simulink model "ctrl_TAPM_2015"  (R2015a)
settings: Solver=ode3  StartTime=0.0  StopTime=inf  FixedStep=0.01  RelTol=1e-3
undefined symbols (not defined in the file): C, D, DiscIntNeverNeededParam, eps_c, epsilon, hd, hd2, I_s, k_cc, K_omega, K_q1f, K_q1r, K_q2f, K_q2r, K_q3f, K_q3r, K_q4f, K_q4r, K_q5f, K_q5r, K_q6f, K_q6r, K_T1f, K_T1r, K_T2f, K_T2r, K_T3f, K_T3r, K_T4f, K_T4r, K_T5f, K_T5r, K_T6f, K_T6r, Kp, Max_Acceleration, Max_rotation, Max_thrust, Min_thrust, n_c, n_max, p_cc, pwm_thr1_backward, pwm_thr1_forward, pwm_thr2_backward, pwm_thr2_forward, pwm_thr3_backward, pwm_thr3_forward, pwm_thr4_backward, pwm_thr4_forward, pwm_thr5_backward, pwm_thr5_forward, pwm_thr6_backward, pwm_thr6_forward, Q_f0, Q_max, r_cc, Rho, Thruster
libraries: marine_gnc x10, dspstat3 x8, simulink x6, simulink_extras x3
(part 5 of 7)

== system ctrl_TAPM_2015/Thruster control /Thruster 3 ==
  Desired thrust 1 : Inport
  shaft speed : Inport  Port=2
  Constant : Constant  Value=hd2.den{1,1}
  Constant1 : Constant  Value=hd2.num{1,1}
  Delay : Delay  DelayLength=1  InitialCondition=0
  Discrete Transfer Fcn : DiscreteTransferFcn  NumeratorSource=Input port  DenominatorSource=Input port  Denominator=[0.2 1]  SampleTime=0.01  a0EqualsOne=on
      settings: InputPortMap=u0,p1,p3
  Losses (placeholder) : Constant  Value=0
  Propeller Hydrodynamics : Subsystem
  Shaft dynamics : Subsystem
  Thruster control : Subsystem
  "Commanded thrust " : Outport
  Shaft speed : Outport  Port=2
  wires:
  Losses (placeholder)/1 -> Propeller Hydrodynamics/1(env)
  Shaft dynamics/1(n) -> Propeller Hydrodynamics/2(n), Shaft speed/1
  Propeller Hydrodynamics/2(Qa) -> Delay/1
  Thruster control/1(Qc) -> Discrete Transfer Fcn/1
  Discrete Transfer Fcn/1 -> Shaft dynamics/1(Qm)
  Desired thrust 1/1 -> Thruster control/1("T_d ")
  Propeller Hydrodynamics/1(Ta) -> "Commanded thrust "/1
  Constant1/1 -> Discrete Transfer Fcn/2
  Constant/1 -> Discrete Transfer Fcn/3
  shaft speed/1 -> Thruster control/2(n)
  Delay/1 -> Shaft dynamics/2(Qa)

== system ctrl_TAPM_2015/Thruster control /Thruster 4 ==
  Desired thrust 1 : Inport
  shaft speed : Inport  Port=2
  Constant : Constant  Value=hd2.den{1,1}
  Constant1 : Constant  Value=hd2.num{1,1}
  Delay : Delay  DelayLength=1  InitialCondition=0
  Discrete Transfer Fcn : DiscreteTransferFcn  NumeratorSource=Input port  DenominatorSource=Input port  Denominator=[0.2 1]  SampleTime=0.01  a0EqualsOne=on
      settings: InputPortMap=u0,p1,p3
  Losses (placeholder) : Constant  Value=0
  Propeller Hydrodynamics : Subsystem
  Shaft dynamics : Subsystem
  Thruster control : Subsystem
  "Commanded thrust " : Outport
  Shaft speed : Outport  Port=2
  wires:
  Losses (placeholder)/1 -> Propeller Hydrodynamics/1(env)
  Shaft dynamics/1(n) -> Propeller Hydrodynamics/2(n), Shaft speed/1
  Propeller Hydrodynamics/2(Qa) -> Delay/1
  Thruster control/1(Qc) -> Discrete Transfer Fcn/1
  Discrete Transfer Fcn/1 -> Shaft dynamics/1(Qm)
  Desired thrust 1/1 -> Thruster control/1("T_d ")
  Propeller Hydrodynamics/1(Ta) -> "Commanded thrust "/1
  Constant1/1 -> Discrete Transfer Fcn/2
  Constant/1 -> Discrete Transfer Fcn/3
  shaft speed/1 -> Thruster control/2(n)
  Delay/1 -> Shaft dynamics/2(Qa)

== system ctrl_TAPM_2015/Thruster control /Thruster 5 ==
  Desired thrust 1 : Inport
  shaft speed : Inport  Port=2
  Constant : Constant  Value=hd2.den{1,1}
  Constant1 : Constant  Value=hd2.num{1,1}
  Delay : Delay  DelayLength=1  InitialCondition=0
  Discrete Transfer Fcn : DiscreteTransferFcn  NumeratorSource=Input port  DenominatorSource=Input port  Denominator=[0.2 1]  SampleTime=0.01  a0EqualsOne=on
      settings: InputPortMap=u0,p1,p3
  Losses (placeholder) : Constant  Value=0
  Propeller Hydrodynamics : Subsystem
  Shaft dynamics : Subsystem
  Thruster control : Subsystem
  "Commanded thrust " : Outport
  Shaft speed : Outport  Port=2
  wires:
  Losses (placeholder)/1 -> Propeller Hydrodynamics/1(env)
  Shaft dynamics/1(n) -> Propeller Hydrodynamics/2(n), Shaft speed/1
  Propeller Hydrodynamics/2(Qa) -> Delay/1
  Thruster control/1(Qc) -> Discrete Transfer Fcn/1
  Discrete Transfer Fcn/1 -> Shaft dynamics/1(Qm)
  Desired thrust 1/1 -> Thruster control/1("T_d ")
  Propeller Hydrodynamics/1(Ta) -> "Commanded thrust "/1
  Constant1/1 -> Discrete Transfer Fcn/2
  Constant/1 -> Discrete Transfer Fcn/3
  shaft speed/1 -> Thruster control/2(n)
  Delay/1 -> Shaft dynamics/2(Qa)

== system ctrl_TAPM_2015/Thruster control /Thruster 6 ==
  Desired thrust 1 : Inport
  shaft speed : Inport  Port=2
  Constant : Constant  Value=hd2.den{1,1}
  Constant1 : Constant  Value=hd2.num{1,1}
  Delay : Delay  DelayLength=1  InitialCondition=0
  Discrete Transfer Fcn : DiscreteTransferFcn  NumeratorSource=Input port  DenominatorSource=Input port  Denominator=[0.2 1]  SampleTime=0.01  a0EqualsOne=on
      settings: InputPortMap=u0,p1,p3
  Losses (placeholder) : Constant  Value=0
  Propeller Hydrodynamics : Subsystem
  Shaft dynamics : Subsystem
  Thruster control : Subsystem
  "Commanded thrust " : Outport
  Shaft speed : Outport  Port=2
  wires:
  Losses (placeholder)/1 -> Propeller Hydrodynamics/1(env)
  Shaft dynamics/1(n) -> Propeller Hydrodynamics/2(n), Shaft speed/1
  Propeller Hydrodynamics/2(Qa) -> Delay/1
  Thruster control/1(Qc) -> Discrete Transfer Fcn/1
  Discrete Transfer Fcn/1 -> Shaft dynamics/1(Qm)
  Desired thrust 1/1 -> Thruster control/1("T_d ")
  Propeller Hydrodynamics/1(Ta) -> "Commanded thrust "/1
  Constant1/1 -> Discrete Transfer Fcn/2
  Constant/1 -> Discrete Transfer Fcn/3
  shaft speed/1 -> Thruster control/2(n)
  Delay/1 -> Shaft dynamics/2(Qa)

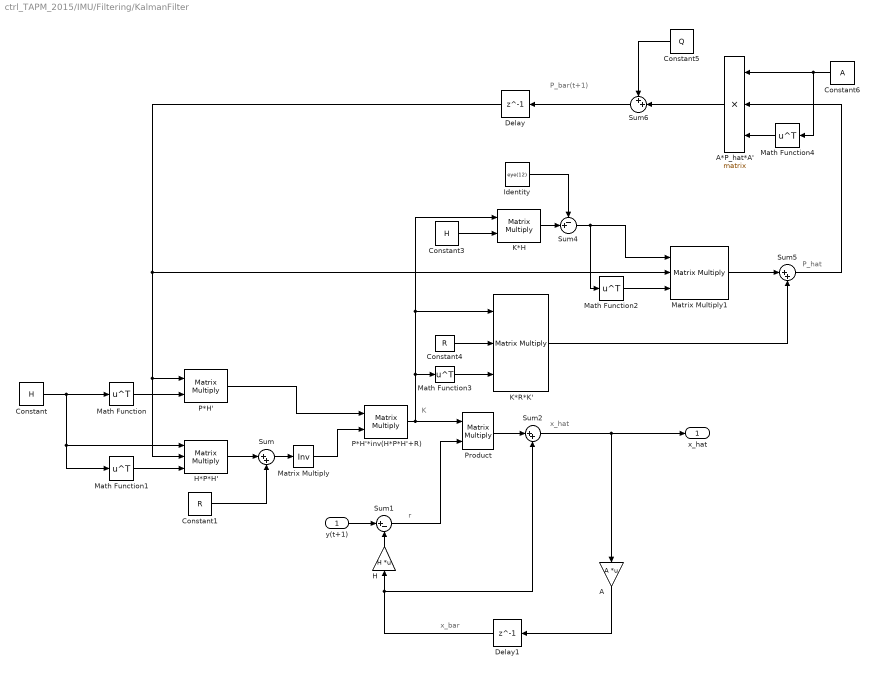
== system ctrl_TAPM_2015/IMU/Filtering/KalmanFilter ==
  note: P_bar(t+1)
  note: P_hat
  note: x_hat
  note: x_bar
  note: r
  note: K
  y(t+1) : Inport
  A : Gain  Gain=A  Multiplication=Matrix(K*u)
  A*P_hat*A' : Product  Inputs=3  Multiplication=Matrix(*)
  Constant : Constant  Value=H
  Constant1 : Constant  Value=R
  Constant3 : Constant  Value=H
  Constant4 : Constant  Value=R
  Constant5 : Constant  Value=Q
  Constant6 : Constant  Value=A
  Delay : Delay  DelayLength=1  InitialCondition=eye(12)
  Delay1 : Delay  DelayLength=1  InitialCondition=[0 0 0 0 0 0 0 0 0 0 0 0]
  H : Gain  Gain=H  Multiplication=Matrix(K*u)
  H*P*H' : Product  Inputs=3  Multiplication=Matrix(*)
  Identity : Constant  Value=eye(12)
  K*H : Product  Multiplication=Matrix(*)
  K*R*K' : Product  Inputs=3  Multiplication=Matrix(*)
  Math Function{,1..4} (5 alike) : Math  Operator=transpose  SaturateOnIntegerOverflow=on
  Matrix Multiply : Product  Inputs=/  Multiplication=Matrix(*)
  Matrix Multiply1 : Product  Inputs=3  Multiplication=Matrix(*)
  P*H' : Product  Multiplication=Matrix(*)
  P*H'*inv(H*P*H'+R) : Product  Multiplication=Matrix(*)
  Product : Product  Multiplication=Matrix(*)
  Sum : Sum  Inputs=|++
  Sum1 : Sum  Inputs=|+-
  Sum2 : Sum  Inputs=|++
  Sum4 : Sum  Inputs=-+|
  Sum5 : Sum  Inputs=|++
  Sum6 : Sum  Inputs=++|
  x_hat : Outport
  wires:
  Constant/1 -> Math Function1/1, H*P*H'/1, Math Function/1
  Math Function/1 -> P*H'/2
  Math Function1/1 -> H*P*H'/3
  H*P*H'/1 -> Sum/1
  Constant1/1 -> Sum/2
  Sum/1 -> Matrix Multiply/1
  Matrix Multiply/1 -> P*H'*inv(H*P*H'+R)/2
  P*H'/1 -> P*H'*inv(H*P*H'+R)/1
  y(t+1)/1 -> Sum1/1
  H/1 -> Sum1/2
  Delay1/1 -> Sum2/2, H/1
  Sum1/1 -> Product/2
  P*H'*inv(H*P*H'+R)/1 -> K*H/1, K*R*K'/1, Math Function3/1, Product/1
  Product/1 -> Sum2/1
  Sum2/1 -> A/1, x_hat/1
  A/1 -> Delay1/1
  Identity/1 -> Sum4/1
  K*H/1 -> Sum4/2
  Constant3/1 -> K*H/2
  Sum4/1 -> Math Function2/1, Matrix Multiply1/1
  Math Function2/1 -> Matrix Multiply1/3
  Constant4/1 -> K*R*K'/2
  Math Function3/1 -> K*R*K'/3
  K*R*K'/1 -> Sum5/2
  Matrix Multiply1/1 -> Sum5/1
  Sum5/1 -> A*P_hat*A'/2
  Sum6/1 -> Delay/1
  Constant5/1 -> Sum6/1
  A*P_hat*A'/1 -> Sum6/2
  Constant6/1 -> Math Function4/1, A*P_hat*A'/1
  Math Function4/1 -> A*P_hat*A'/3
  Delay/1 -> H*P*H'/2, P*H'/1, Matrix Multiply1/2

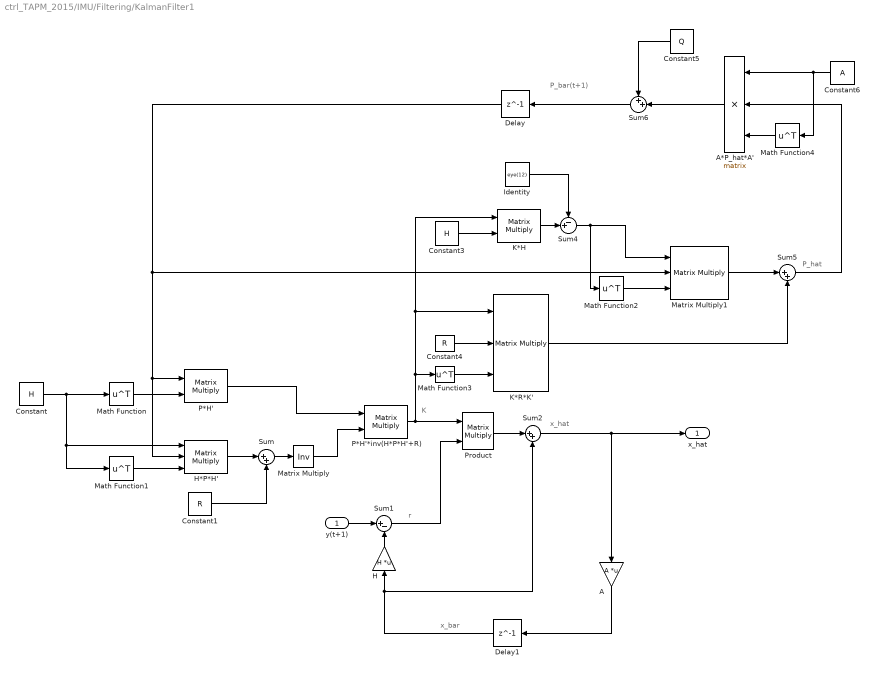
== system ctrl_TAPM_2015/IMU/Filtering/KalmanFilter1 ==
  note: P_bar(t+1)
  note: P_hat
  note: x_hat
  note: x_bar
  note: r
  note: K
  y(t+1) : Inport
  A : Gain  Gain=A  Multiplication=Matrix(K*u)
  A*P_hat*A' : Product  Inputs=3  Multiplication=Matrix(*)
  Constant : Constant  Value=H
  Constant1 : Constant  Value=R
  Constant3 : Constant  Value=H
  Constant4 : Constant  Value=R
  Constant5 : Constant  Value=Q
  Constant6 : Constant  Value=A
  Delay : Delay  DelayLength=1  InitialCondition=eye(12)
  Delay1 : Delay  DelayLength=1  InitialCondition=[0 0 0 0 0 0 0 0 0 0 0 0]
  H : Gain  Gain=H  Multiplication=Matrix(K*u)
  H*P*H' : Product  Inputs=3  Multiplication=Matrix(*)
  Identity : Constant  Value=eye(12)
  K*H : Product  Multiplication=Matrix(*)
  K*R*K' : Product  Inputs=3  Multiplication=Matrix(*)
  Math Function{,1..4} (5 alike) : Math  Operator=transpose  SaturateOnIntegerOverflow=on
  Matrix Multiply : Product  Inputs=/  Multiplication=Matrix(*)
  Matrix Multiply1 : Product  Inputs=3  Multiplication=Matrix(*)
  P*H' : Product  Multiplication=Matrix(*)
  P*H'*inv(H*P*H'+R) : Product  Multiplication=Matrix(*)
  Product : Product  Multiplication=Matrix(*)
  Sum : Sum  Inputs=|++
  Sum1 : Sum  Inputs=|+-
  Sum2 : Sum  Inputs=|++
  Sum4 : Sum  Inputs=-+|
  Sum5 : Sum  Inputs=|++
  Sum6 : Sum  Inputs=++|
  x_hat : Outport
  wires:
  Constant/1 -> Math Function1/1, H*P*H'/1, Math Function/1
  Math Function/1 -> P*H'/2
  Math Function1/1 -> H*P*H'/3
  H*P*H'/1 -> Sum/1
  Constant1/1 -> Sum/2
  Sum/1 -> Matrix Multiply/1
  Matrix Multiply/1 -> P*H'*inv(H*P*H'+R)/2
  P*H'/1 -> P*H'*inv(H*P*H'+R)/1
  y(t+1)/1 -> Sum1/1
  H/1 -> Sum1/2
  Delay1/1 -> Sum2/2, H/1
  Sum1/1 -> Product/2
  P*H'*inv(H*P*H'+R)/1 -> K*H/1, K*R*K'/1, Math Function3/1, Product/1
  Product/1 -> Sum2/1
  Sum2/1 -> A/1, x_hat/1
  A/1 -> Delay1/1
  Identity/1 -> Sum4/1
  K*H/1 -> Sum4/2
  Constant3/1 -> K*H/2
  Sum4/1 -> Math Function2/1, Matrix Multiply1/1
  Math Function2/1 -> Matrix Multiply1/3
  Constant4/1 -> K*R*K'/2
  Math Function3/1 -> K*R*K'/3
  K*R*K'/1 -> Sum5/2
  Matrix Multiply1/1 -> Sum5/1
  Sum5/1 -> A*P_hat*A'/2
  Sum6/1 -> Delay/1
  Constant5/1 -> Sum6/1
  A*P_hat*A'/1 -> Sum6/2
  Constant6/1 -> Math Function4/1, A*P_hat*A'/1
  Math Function4/1 -> A*P_hat*A'/3
  Delay/1 -> H*P*H'/2, P*H'/1, Matrix Multiply1/2

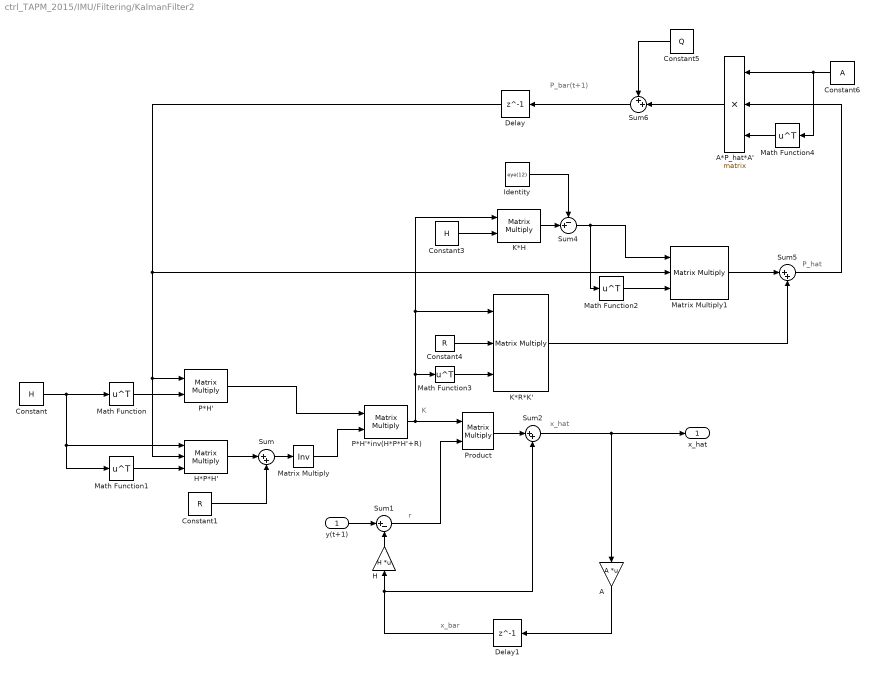
== system ctrl_TAPM_2015/IMU/Filtering/KalmanFilter2 ==
  note: P_bar(t+1)
  note: P_hat
  note: x_hat
  note: x_bar
  note: r
  note: K
  y(t+1) : Inport
  A : Gain  Gain=A  Multiplication=Matrix(K*u)
  A*P_hat*A' : Product  Inputs=3  Multiplication=Matrix(*)
  Constant : Constant  Value=H
  Constant1 : Constant  Value=R
  Constant3 : Constant  Value=H
  Constant4 : Constant  Value=R
  Constant5 : Constant  Value=Q
  Constant6 : Constant  Value=A
  Delay : Delay  DelayLength=1  InitialCondition=eye(12)
  Delay1 : Delay  DelayLength=1  InitialCondition=[0 0 0 0 0 0 0 0 0 0 0 0]
  H : Gain  Gain=H  Multiplication=Matrix(K*u)
  H*P*H' : Product  Inputs=3  Multiplication=Matrix(*)
  Identity : Constant  Value=eye(12)
  K*H : Product  Multiplication=Matrix(*)
  K*R*K' : Product  Inputs=3  Multiplication=Matrix(*)
  Math Function{,1..4} (5 alike) : Math  Operator=transpose  SaturateOnIntegerOverflow=on
  Matrix Multiply : Product  Inputs=/  Multiplication=Matrix(*)
  Matrix Multiply1 : Product  Inputs=3  Multiplication=Matrix(*)
  P*H' : Product  Multiplication=Matrix(*)
  P*H'*inv(H*P*H'+R) : Product  Multiplication=Matrix(*)
  Product : Product  Multiplication=Matrix(*)
  Sum : Sum  Inputs=|++
  Sum1 : Sum  Inputs=|+-
  Sum2 : Sum  Inputs=|++
  Sum4 : Sum  Inputs=-+|
  Sum5 : Sum  Inputs=|++
  Sum6 : Sum  Inputs=++|
  x_hat : Outport
  wires:
  Constant/1 -> Math Function1/1, H*P*H'/1, Math Function/1
  Math Function/1 -> P*H'/2
  Math Function1/1 -> H*P*H'/3
  H*P*H'/1 -> Sum/1
  Constant1/1 -> Sum/2
  Sum/1 -> Matrix Multiply/1
  Matrix Multiply/1 -> P*H'*inv(H*P*H'+R)/2
  P*H'/1 -> P*H'*inv(H*P*H'+R)/1
  y(t+1)/1 -> Sum1/1
  H/1 -> Sum1/2
  Delay1/1 -> Sum2/2, H/1
  Sum1/1 -> Product/2
  P*H'*inv(H*P*H'+R)/1 -> K*H/1, K*R*K'/1, Math Function3/1, Product/1
  Product/1 -> Sum2/1
  Sum2/1 -> A/1, x_hat/1
  A/1 -> Delay1/1
  Identity/1 -> Sum4/1
  K*H/1 -> Sum4/2
  Constant3/1 -> K*H/2
  Sum4/1 -> Math Function2/1, Matrix Multiply1/1
  Math Function2/1 -> Matrix Multiply1/3
  Constant4/1 -> K*R*K'/2
  Math Function3/1 -> K*R*K'/3
  K*R*K'/1 -> Sum5/2
  Matrix Multiply1/1 -> Sum5/1
  Sum5/1 -> A*P_hat*A'/2
  Sum6/1 -> Delay/1
  Constant5/1 -> Sum6/1
  A*P_hat*A'/1 -> Sum6/2
  Constant6/1 -> Math Function4/1, A*P_hat*A'/1
  Math Function4/1 -> A*P_hat*A'/3
  Delay/1 -> H*P*H'/2, P*H'/1, Matrix Multiply1/2

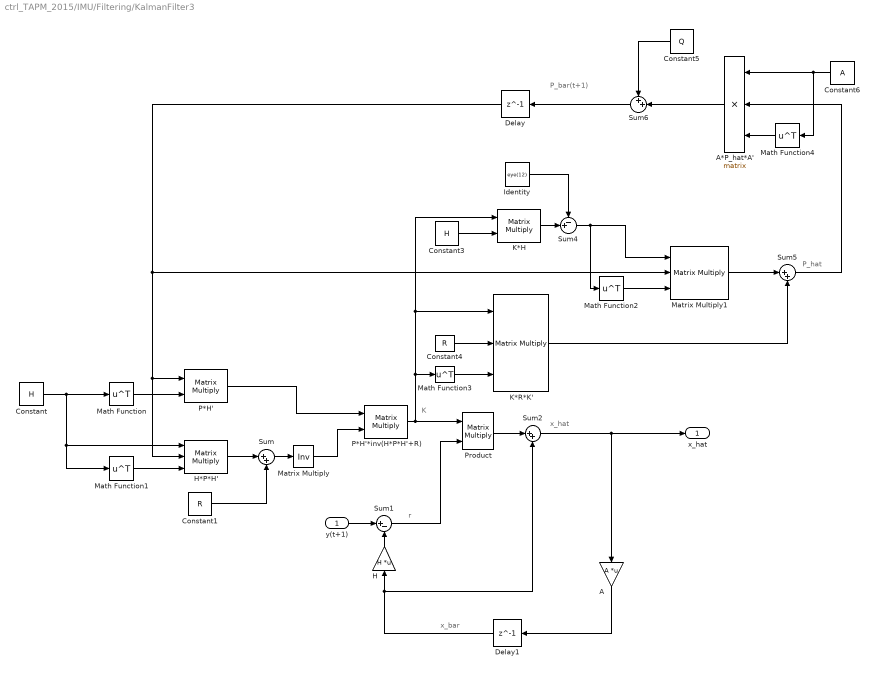
== system ctrl_TAPM_2015/IMU/Filtering/KalmanFilter3 ==
  note: P_bar(t+1)
  note: P_hat
  note: x_hat
  note: x_bar
  note: r
  note: K
  y(t+1) : Inport
  A : Gain  Gain=A  Multiplication=Matrix(K*u)
  A*P_hat*A' : Product  Inputs=3  Multiplication=Matrix(*)
  Constant : Constant  Value=H
  Constant1 : Constant  Value=R
  Constant3 : Constant  Value=H
  Constant4 : Constant  Value=R
  Constant5 : Constant  Value=Q
  Constant6 : Constant  Value=A
  Delay : Delay  DelayLength=1  InitialCondition=eye(12)
  Delay1 : Delay  DelayLength=1  InitialCondition=[0 0 0 0 0 0 0 0 0 0 0 0]
  H : Gain  Gain=H  Multiplication=Matrix(K*u)
  H*P*H' : Product  Inputs=3  Multiplication=Matrix(*)
  Identity : Constant  Value=eye(12)
  K*H : Product  Multiplication=Matrix(*)
  K*R*K' : Product  Inputs=3  Multiplication=Matrix(*)
  Math Function{,1..4} (5 alike) : Math  Operator=transpose  SaturateOnIntegerOverflow=on
  Matrix Multiply : Product  Inputs=/  Multiplication=Matrix(*)
  Matrix Multiply1 : Product  Inputs=3  Multiplication=Matrix(*)
  P*H' : Product  Multiplication=Matrix(*)
  P*H'*inv(H*P*H'+R) : Product  Multiplication=Matrix(*)
  Product : Product  Multiplication=Matrix(*)
  Sum : Sum  Inputs=|++
  Sum1 : Sum  Inputs=|+-
  Sum2 : Sum  Inputs=|++
  Sum4 : Sum  Inputs=-+|
  Sum5 : Sum  Inputs=|++
  Sum6 : Sum  Inputs=++|
  x_hat : Outport
  wires:
  Constant/1 -> Math Function1/1, H*P*H'/1, Math Function/1
  Math Function/1 -> P*H'/2
  Math Function1/1 -> H*P*H'/3
  H*P*H'/1 -> Sum/1
  Constant1/1 -> Sum/2
  Sum/1 -> Matrix Multiply/1
  Matrix Multiply/1 -> P*H'*inv(H*P*H'+R)/2
  P*H'/1 -> P*H'*inv(H*P*H'+R)/1
  y(t+1)/1 -> Sum1/1
  H/1 -> Sum1/2
  Delay1/1 -> Sum2/2, H/1
  Sum1/1 -> Product/2
  P*H'*inv(H*P*H'+R)/1 -> K*H/1, K*R*K'/1, Math Function3/1, Product/1
  Product/1 -> Sum2/1
  Sum2/1 -> A/1, x_hat/1
  A/1 -> Delay1/1
  Identity/1 -> Sum4/1
  K*H/1 -> Sum4/2
  Constant3/1 -> K*H/2
  Sum4/1 -> Math Function2/1, Matrix Multiply1/1
  Math Function2/1 -> Matrix Multiply1/3
  Constant4/1 -> K*R*K'/2
  Math Function3/1 -> K*R*K'/3
  K*R*K'/1 -> Sum5/2
  Matrix Multiply1/1 -> Sum5/1
  Sum5/1 -> A*P_hat*A'/2
  Sum6/1 -> Delay/1
  Constant5/1 -> Sum6/1
  A*P_hat*A'/1 -> Sum6/2
  Constant6/1 -> Math Function4/1, A*P_hat*A'/1
  Math Function4/1 -> A*P_hat*A'/3
  Delay/1 -> H*P*H'/2, P*H'/1, Matrix Multiply1/2

== system ctrl_TAPM_2015/IMU/Filtering/Outliner cleaner ==
  Y : Inport
  Abs : Abs
  Abs1 : Abs
  Gain : Gain  Gain=2*1.4826
  If : If  NumInputs=2  IfExpression=u1 < u2
  Median : dspstat3/Median  sortAlg=Quick sort  directionMode=Entire input  dimension=1  outputDataTypeStr=Inherit: Same as accumulator  outputLastDataTypeStr=Inherit: Same as accumulator  outputMin=[]  outputMax=[]  accumDataTypeStr=Inherit: Same as product output  accumLastDataTypeStr=Inherit: Same as product output  roundingMode=Floor  overflowMode=off  treatSBRowAsCol=off
      settings: allowOverrides=off
  Median1 : dspstat3/Median  sortAlg=Quick sort  directionMode=Entire input  dimension=1  outputDataTypeStr=Inherit: Same as accumulator  outputLastDataTypeStr=Inherit: Same as accumulator  outputMin=[]  outputMax=[]  accumDataTypeStr=Inherit: Same as product output  accumLastDataTypeStr=Inherit: Same as product output  roundingMode=Floor  overflowMode=off  treatSBRowAsCol=off
      settings: allowOverrides=off
  Memory2 : Memory  X0=[4.968, 4.965, 4.97, 4.975, 4.96]
  Memory3 : Memory  X0=[0, 0, 0, 0, 0, 0, 0]
  Merge : Merge
  Merge1 : Merge
  No outlier : Subsystem  TreatAsAtomicUnit=on
  Outlier detected : Subsystem  TreatAsAtomicUnit=on
  Selector : Selector  InputPortWidth=7  IndexOptions=Index vector (dialog)  Indices=[7]  OutputSizes=1
  Sum : Sum  Inputs=+-|
  Sum1 : Sum  Inputs=-+|
  Y2 : InportShadow
  Y_filtered : Outport
  wires:
  Memory2/1 -> Sum/1, [V_old], Median/1
  Median/1 -> Sum1/1, Sum/2
  Sum/1 -> Abs/1
  Abs/1 -> Median1/1
  Y/1 -> Memory3/1, Selector/1
  Selector/1 -> Sum1/2
  Sum1/1 -> Abs1/1
  Abs1/1 -> If/2
  Gain/1 -> If/1
  [Y_prev] -> Outlier detected/1(Y_previous)
  Outlier detected/1(Y_filtered) -> Merge/1
  If/1 -> Outlier detected/Action
  If/2 -> No outlier/Action
  Y2/1 -> No outlier/1(Y)
  Merge1/1 -> Memory2/1
  No outlier/1(Y_filtered) -> Merge/2
  Median1/1 -> Gain/1
  Memory3/1 -> [Y_prev]
  Merge/1 -> Y_filtered/1
  [V_old] -> Outlier detected/2(V)
  Outlier detected/2(V_hist) -> Merge1/1
  [V_old] -> No outlier/2(V)
  No outlier/2(V_hist) -> Merge1/2

== system ctrl_TAPM_2015/IMU/Filtering/Outliner cleaner1 ==
  Y : Inport
  Abs : Abs
  Abs1 : Abs
  Gain : Gain  Gain=2*1.4826
  If : If  NumInputs=2  IfExpression=u1 < u2
  Median : dspstat3/Median  sortAlg=Quick sort  directionMode=Entire input  dimension=1  outputDataTypeStr=Inherit: Same as accumulator  outputLastDataTypeStr=Inherit: Same as accumulator  outputMin=[]  outputMax=[]  accumDataTypeStr=Inherit: Same as product output  accumLastDataTypeStr=Inherit: Same as product output  roundingMode=Floor  overflowMode=off  treatSBRowAsCol=off
      settings: allowOverrides=off
  Median1 : dspstat3/Median  sortAlg=Quick sort  directionMode=Entire input  dimension=1  outputDataTypeStr=Inherit: Same as accumulator  outputLastDataTypeStr=Inherit: Same as accumulator  outputMin=[]  outputMax=[]  accumDataTypeStr=Inherit: Same as product output  accumLastDataTypeStr=Inherit: Same as product output  roundingMode=Floor  overflowMode=off  treatSBRowAsCol=off
      settings: allowOverrides=off
  Memory2 : Memory  X0=[4.968, 4.965, 4.97, 4.975, 4.96]
  Memory3 : Memory  X0=[0, 0, 0, 0, 0, 0, 0]
  Merge : Merge
  Merge1 : Merge
  No outlier : Subsystem  TreatAsAtomicUnit=on
  Outlier detected : Subsystem  TreatAsAtomicUnit=on
  Selector : Selector  InputPortWidth=7  IndexOptions=Index vector (dialog)  Indices=[7]  OutputSizes=1
  Sum : Sum  Inputs=+-|
  Sum1 : Sum  Inputs=-+|
  Y2 : InportShadow
  Y_filtered : Outport
  wires:
  Memory2/1 -> Sum/1, [V_old], Median/1
  Median/1 -> Sum1/1, Sum/2
  Sum/1 -> Abs/1
  Abs/1 -> Median1/1
  Y/1 -> Memory3/1, Selector/1
  Selector/1 -> Sum1/2
  Sum1/1 -> Abs1/1
  Abs1/1 -> If/2
  Gain/1 -> If/1
  [Y_prev] -> Outlier detected/1(Y_previous)
  Outlier detected/1(Y_filtered) -> Merge/1
  If/1 -> Outlier detected/Action
  If/2 -> No outlier/Action
  Y2/1 -> No outlier/1(Y)
  Merge1/1 -> Memory2/1
  No outlier/1(Y_filtered) -> Merge/2
  Median1/1 -> Gain/1
  Memory3/1 -> [Y_prev]
  Merge/1 -> Y_filtered/1
  [V_old] -> Outlier detected/2(V)
  Outlier detected/2(V_hist) -> Merge1/1
  [V_old] -> No outlier/2(V)
  No outlier/2(V_hist) -> Merge1/2

== system ctrl_TAPM_2015/IMU/Filtering/Outliner cleaner2 ==
  Y : Inport
  Abs : Abs
  Abs1 : Abs
  Gain : Gain  Gain=2*1.4826
  If : If  NumInputs=2  IfExpression=u1 < u2
  Median : dspstat3/Median  sortAlg=Quick sort  directionMode=Entire input  dimension=1  outputDataTypeStr=Inherit: Same as accumulator  outputLastDataTypeStr=Inherit: Same as accumulator  outputMin=[]  outputMax=[]  accumDataTypeStr=Inherit: Same as product output  accumLastDataTypeStr=Inherit: Same as product output  roundingMode=Floor  overflowMode=off  treatSBRowAsCol=off
      settings: allowOverrides=off
  Median1 : dspstat3/Median  sortAlg=Quick sort  directionMode=Entire input  dimension=1  outputDataTypeStr=Inherit: Same as accumulator  outputLastDataTypeStr=Inherit: Same as accumulator  outputMin=[]  outputMax=[]  accumDataTypeStr=Inherit: Same as product output  accumLastDataTypeStr=Inherit: Same as product output  roundingMode=Floor  overflowMode=off  treatSBRowAsCol=off
      settings: allowOverrides=off
  Memory2 : Memory  X0=[4.968, 4.965, 4.97, 4.975, 4.96]
  Memory3 : Memory  X0=[0, 0, 0, 0, 0, 0, 0]
  Merge : Merge
  Merge1 : Merge
  No outlier : Subsystem  TreatAsAtomicUnit=on
  Outlier detected : Subsystem  TreatAsAtomicUnit=on
  Selector : Selector  InputPortWidth=7  IndexOptions=Index vector (dialog)  Indices=[7]  OutputSizes=1
  Sum : Sum  Inputs=+-|
  Sum1 : Sum  Inputs=-+|
  Y2 : InportShadow
  Y_filtered : Outport
  wires:
  Memory2/1 -> Sum/1, [V_old], Median/1
  Median/1 -> Sum1/1, Sum/2
  Sum/1 -> Abs/1
  Abs/1 -> Median1/1
  Y/1 -> Memory3/1, Selector/1
  Selector/1 -> Sum1/2
  Sum1/1 -> Abs1/1
  Abs1/1 -> If/2
  Gain/1 -> If/1
  [Y_prev] -> Outlier detected/1(Y_previous)
  Outlier detected/1(Y_filtered) -> Merge/1
  If/1 -> Outlier detected/Action
  If/2 -> No outlier/Action
  Y2/1 -> No outlier/1(Y)
  Merge1/1 -> Memory2/1
  No outlier/1(Y_filtered) -> Merge/2
  Median1/1 -> Gain/1
  Memory3/1 -> [Y_prev]
  Merge/1 -> Y_filtered/1
  [V_old] -> Outlier detected/2(V)
  Outlier detected/2(V_hist) -> Merge1/1
  [V_old] -> No outlier/2(V)
  No outlier/2(V_hist) -> Merge1/2

== system ctrl_TAPM_2015/IMU/Filtering/Outliner cleaner3 ==
  Y : Inport
  Abs : Abs
  Abs1 : Abs
  Gain : Gain  Gain=2*1.4826
  If : If  NumInputs=2  IfExpression=u1 < u2
  Median : dspstat3/Median  sortAlg=Quick sort  directionMode=Entire input  dimension=1  outputDataTypeStr=Inherit: Same as accumulator  outputLastDataTypeStr=Inherit: Same as accumulator  outputMin=[]  outputMax=[]  accumDataTypeStr=Inherit: Same as product output  accumLastDataTypeStr=Inherit: Same as product output  roundingMode=Floor  overflowMode=off  treatSBRowAsCol=off
      settings: allowOverrides=off
  Median1 : dspstat3/Median  sortAlg=Quick sort  directionMode=Entire input  dimension=1  outputDataTypeStr=Inherit: Same as accumulator  outputLastDataTypeStr=Inherit: Same as accumulator  outputMin=[]  outputMax=[]  accumDataTypeStr=Inherit: Same as product output  accumLastDataTypeStr=Inherit: Same as product output  roundingMode=Floor  overflowMode=off  treatSBRowAsCol=off
      settings: allowOverrides=off
  Memory2 : Memory  X0=[4.968, 4.965, 4.97, 4.975, 4.96]
  Memory3 : Memory  X0=[0, 0, 0, 0, 0, 0, 0]
  Merge : Merge
  Merge1 : Merge
  No outlier : Subsystem  TreatAsAtomicUnit=on
  Outlier detected : Subsystem  TreatAsAtomicUnit=on
  Selector : Selector  InputPortWidth=7  IndexOptions=Index vector (dialog)  Indices=[7]  OutputSizes=1
  Sum : Sum  Inputs=+-|
  Sum1 : Sum  Inputs=-+|
  Y2 : InportShadow
  Y_filtered : Outport
  wires:
  Memory2/1 -> Sum/1, [V_old], Median/1
  Median/1 -> Sum1/1, Sum/2
  Sum/1 -> Abs/1
  Abs/1 -> Median1/1
  Y/1 -> Memory3/1, Selector/1
  Selector/1 -> Sum1/2
  Sum1/1 -> Abs1/1
  Abs1/1 -> If/2
  Gain/1 -> If/1
  [Y_prev] -> Outlier detected/1(Y_previous)
  Outlier detected/1(Y_filtered) -> Merge/1
  If/1 -> Outlier detected/Action
  If/2 -> No outlier/Action
  Y2/1 -> No outlier/1(Y)
  Merge1/1 -> Memory2/1
  No outlier/1(Y_filtered) -> Merge/2
  Median1/1 -> Gain/1
  Memory3/1 -> [Y_prev]
  Merge/1 -> Y_filtered/1
  [V_old] -> Outlier detected/2(V)
  Outlier detected/2(V_hist) -> Merge1/1
  [V_old] -> No outlier/2(V)
  No outlier/2(V_hist) -> Merge1/2

== system ctrl_TAPM_2015/TAPM Controller w_observer/PID/DP controller ==
  eta_ref : Inport
  eta : Inport  Port=2
  nu : Inport  Port=3
  Demux : Demux  Outputs=3
  Integrator : Integrator
  Matrix Multiply : Product  Multiplication=Matrix(*)
  Matrix Multiply1 : Product  Multiplication=Matrix(*)
  Matrix Multiply2 : Product  Multiplication=Matrix(*)
  Mux : Mux  Inputs=3
  Sum1 : Sum  Inputs=|+-  SaturateOnIntegerOverflow=on  InputSameDT=on  OutDataTypeStr=Inherit: Same as first input
  Sum2 : Sum  Inputs=+-|  SaturateOnIntegerOverflow=on  InputSameDT=on  OutDataTypeStr=Inherit: Same as first input
  Sum3 : Sum  Inputs=|++  SaturateOnIntegerOverflow=on  InputSameDT=on  OutDataTypeStr=Inherit: Same as first input
  Transposed rotation matrix in yaw1 : marine_gnc/Models/ Kinematics/Transposed rotation  matrix in yaw
  "[-inf inf] to [-pi pi]" : marine_gnc/Utilities/Math Operations/[-inf inf] to [-pi pi]
  "[-inf inf] to [-pi pi]1" : marine_gnc/Utilities/Math Operations/[-inf inf] to [-pi pi]
  yaw angle : Fcn  Expr=u(3)
  tau : Outport  InitialOutput=0
  wires:
  "[-inf inf] to [-pi pi]1"/1 -> Transposed rotation matrix in yaw1/1
  yaw angle/1 -> "[-inf inf] to [-pi pi]1"/1  "psi"
  Mux/1 -> Transposed rotation matrix in yaw1/2
  Demux/1 -> Mux/1
  Demux/2 -> Mux/2
  "[-inf inf] to [-pi pi]"/1 -> Mux/3
  Sum2/1 -> Demux/1  "regulation error"
  Demux/3 -> "[-inf inf] to [-pi pi]"/1
  eta_ref/1 -> Sum2/1
  Sum1/1 -> tau/1
  eta/1 -> Sum2/2, yaw angle/1
  nu/1 -> Matrix Multiply2/2
  Matrix Multiply2/1 -> Sum1/2
  Matrix Multiply/1 -> Sum3/1
  Sum3/1 -> Sum1/1
  Matrix Multiply1/1 -> Sum3/2
  Transposed rotation matrix in yaw1/1 -> Matrix Multiply/2, Integrator/1
  [K_p] -> Matrix Multiply/1
  Integrator/1 -> Matrix Multiply1/2
  [K_i] -> Matrix Multiply1/1
  [K_d] -> Matrix Multiply2/1

== system ctrl_TAPM_2015/TAPM Controller w_observer/PID/DP controller1 ==
  eta_ref : Inport
  eta : Inport  Port=2
  nu : Inport  Port=3
  Demux : Demux  Outputs=3
  Integrator : Integrator
  Matrix Multiply : Product  Multiplication=Matrix(*)
  Matrix Multiply1 : Product  Multiplication=Matrix(*)
  Matrix Multiply2 : Product  Multiplication=Matrix(*)
  Mux : Mux  Inputs=3
  Sum1 : Sum  Inputs=|+-  SaturateOnIntegerOverflow=on  InputSameDT=on  OutDataTypeStr=Inherit: Same as first input
  Sum2 : Sum  Inputs=+-|  SaturateOnIntegerOverflow=on  InputSameDT=on  OutDataTypeStr=Inherit: Same as first input
  Sum3 : Sum  Inputs=|++  SaturateOnIntegerOverflow=on  InputSameDT=on  OutDataTypeStr=Inherit: Same as first input
  Transposed rotation matrix in yaw1 : marine_gnc/Models/ Kinematics/Transposed rotation  matrix in yaw
  "[-inf inf] to [-pi pi]" : marine_gnc/Utilities/Math Operations/[-inf inf] to [-pi pi]
  "[-inf inf] to [-pi pi]1" : marine_gnc/Utilities/Math Operations/[-inf inf] to [-pi pi]
  yaw angle : Fcn  Expr=u(3)
  tau : Outport  InitialOutput=0
  wires:
  "[-inf inf] to [-pi pi]1"/1 -> Transposed rotation matrix in yaw1/1
  yaw angle/1 -> "[-inf inf] to [-pi pi]1"/1  "psi"
  Mux/1 -> Transposed rotation matrix in yaw1/2
  Demux/1 -> Mux/1
  Demux/2 -> Mux/2
  "[-inf inf] to [-pi pi]"/1 -> Mux/3
  Sum2/1 -> Demux/1  "regulation error"
  Demux/3 -> "[-inf inf] to [-pi pi]"/1
  eta_ref/1 -> Sum2/1
  Sum1/1 -> tau/1
  eta/1 -> Sum2/2, yaw angle/1
  nu/1 -> Matrix Multiply2/2
  Matrix Multiply2/1 -> Sum1/2
  Matrix Multiply/1 -> Sum3/1
  Sum3/1 -> Sum1/1
  Matrix Multiply1/1 -> Sum3/2
  Transposed rotation matrix in yaw1/1 -> Matrix Multiply/2, Integrator/1
  [K_p_outside] -> Matrix Multiply/1
  Integrator/1 -> Matrix Multiply1/2
  [K_i_outside] -> Matrix Multiply1/1
  [K_d_outside] -> Matrix Multiply2/1

== system ctrl_TAPM_2015/Thruster control /Thruster 1/Propeller Hydrodynamics ==
  env : Inport
  n : Inport  Port=2
  Actual Force and Torque : MATLAB Function  TreatAsAtomicUnit=on
      settings: PermitHierarchicalResolution=ParametersOnly
  Control_test_Pa : S-Function  Priority=1  FunctionName=NIVeriStandIO  Parameters=width dtype portnum stime stype btype  SFunctionDeploymentMode=off  EnableBusSupport=off  mask(NI VeriStand Outport){portnum=1, width=-1, stime=-1, dtype=auto, stype=auto, btype=0}
      mask prompts: portnum "Port number:"; width "Port dimensions (-1 for dynamically sized):"; stime "Sample time (-1 for inherited):"; dtype "Data type:"; stype "Signal type:"; btype "Block type:"
      mask help: Use this outport on any level of nested subsystems to allow NI VeriStand software to map signals to it.
      mask init:
      | NIVeriStandIO_init;
      settings: CopyFcn=NIVeriStand_MDL_functions('', 'IO_copy');  DeleteFcn=NIVeriStand_MDL_functions('', 'IO_delete');  MoveFcn=set_param(gcb, 'Mask', 'on');
      mask Callback portnum: NIVeriStand_MDL_functions('', 'IO_setportnum');
      mask TypeOptions dtype: auto | double | single | int8 | uint8 | int16 | uint16 | int32 | uint32 | boolean
      mask Callback dtype: NIVeriStand_MDL_functions('', 'IO_booleansignal');
      mask TypeOptions stype: auto | real | complex
      mask Display:
      | patch([-x x], [-y y], [.90980 .81960 .32156]);
      | plot([xrad -x x xrad], [yrad -y y yrad]);
      | fprintf('NI Out%d', portnum);
  Ta : Outport
  Qa : Outport  Port=2
  wires:
  n/1 -> Actual Force and Torque/1(n)
  [D] -> Actual Force and Torque/7(D)
  [Kq1f] -> Actual Force and Torque/2(Kq)
  Actual Force and Torque/2(Qa) -> Qa/1
  [Rho] -> Actual Force and Torque/6(Rho)
  env/1 -> Actual Force and Torque/9(env)
  [Kt1f] -> Actual Force and Torque/3(Kt)
  Actual Force and Torque/1(Ta) -> Ta/1
  [Kt1r] -> Actual Force and Torque/4(Ktr)
  [Kq1r] -> Actual Force and Torque/5(Kqr)
  [eps_c] -> Actual Force and Torque/8(eps_c)
  Actual Force and Torque/3(Pa) -> Control_test_Pa/1

== system ctrl_TAPM_2015/Thruster control /Thruster 1/Shaft dynamics ==
  Qm : Inport
  Qa : Inport  Port=2
  Finding rotation speed : Gain  Gain=1/(2*pi*I_s)
  Integrator : Integrator  ExternalReset=either
  K_omega : Gain  Gain=K_omega*2*pi
  Sum : Sum  Inputs=-+-
  reset : S-Function  Priority=1  FunctionName=NIVeriStandIO  Parameters=width dtype portnum stime stype btype  SFunctionDeploymentMode=off  EnableBusSupport=off  mask(NI VeriStand Inport){portnum=1, width=-1, stime=-1, dtype=auto, stype=auto, btype=1}
      mask prompts: portnum "Port number:"; width "Port dimensions (-1 for dynamically sized):"; stime "Sample time (-1 for inherited):"; dtype "Data type:"; stype "Signal type:"; btype "Block type:"
      mask help: Use this inport on any level of nested subsystems to allow NI VeriStand software to map signals to it.
      mask init:
      | NIVeriStandIO_init;
      settings: CopyFcn=NIVeriStand_MDL_functions('', 'IO_copy');  DeleteFcn=NIVeriStand_MDL_functions('', 'IO_delete');  MoveFcn=set_param(gcb, 'Mask', 'on');
      mask Callback portnum: NIVeriStand_MDL_functions('', 'IO_setportnum');
      mask TypeOptions dtype: auto | double | single | int8 | uint8 | int16 | uint16 | int32 | uint32 | boolean
      mask Callback dtype: NIVeriStand_MDL_functions('', 'IO_booleansignal');
      mask TypeOptions stype: auto | real | complex
      mask Display:
      | patch([-x x], [-y y], [.90980 .81960 .32156]);
      | plot([xrad -x x xrad], [yrad -y y yrad]);
      | fprintf('NI In%d', portnum);
  n : Outport
  wires:
  Qm/1 -> Sum/2
  Sum/1 -> Finding rotation speed/1
  Qa/1 -> Sum/1
  K_omega/1 -> Sum/3
  Finding rotation speed/1 -> Integrator/1
  Integrator/1 -> K_omega/1, n/1
  reset/1 -> Integrator/2

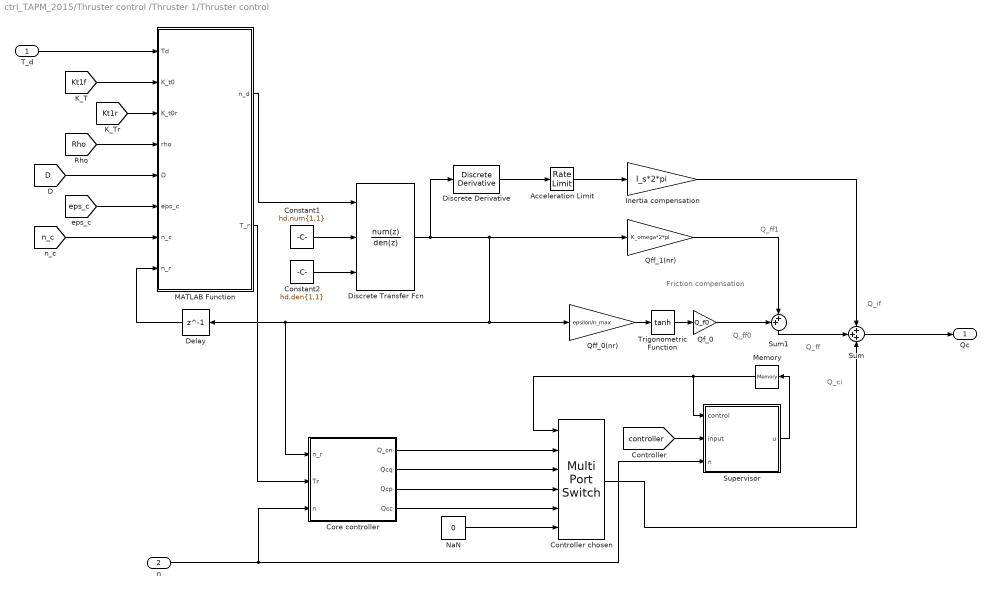
== system ctrl_TAPM_2015/Thruster control /Thruster 1/Thruster control ==
  note: Q_ci
  note: Q_if
  note: Q_ff
  note: Q_ff0
  note: Q_ff1
  note: Friction compensation
  "T_d " : Inport
  n : Inport  Port=2
  Acceleration Limit : RateLimiter  RisingSlewLimit=Max_Acceleration  FallingSlewLimit=-Max_Acceleration  SampleTimeMode=inherited
  Constant1 : Constant  Value=hd.num{1,1}  VectorParams1D=off
  Constant2 : Constant  Value=hd.den{1,1}  VectorParams1D=off
  Controller chosen : MultiPortSwitch  Inputs=5
  Core controller : Subsystem
  Delay : Delay  DelayLength=1  InitialCondition=0
  Discrete Transfer Fcn : DiscreteTransferFcn  NumeratorSource=Input port  Numerator=[8.76e-05 0.0003481 8.648e-05]  DenominatorSource=Input port  Denominator=[1 -1.974 0.9746]  SampleTime=0.01  a0EqualsOne=on
      settings: InputPortMap=u0,p1,p3
  Discrete Derivative : simulink/Discrete/Discrete Derivative  gainval=1.0  ICPrevScaledInput=0.0  InputProcessing=Inherited  OutMin=[]  OutMax=[]  OutDataType=fixdt(1, 16)  OutScaling=2^-10  DoSatur=off
  Inertia compensation : Gain  Gain=I_s*2*pi
  MATLAB Function : MATLAB Function  TreatAsAtomicUnit=on
      settings: PermitHierarchicalResolution=ParametersOnly
  Memory : Memory  X0=1  InheritSampleTime=on
  NaN : Constant  Value=0
  Qf_0 : Gain  Gain=Q_f0
  Qff_0(nr) : Gain  Gain=epsilon/n_max
  Qff_1(nr) : Gain  Gain=K_omega*2*pi
  Sum : Sum  Inputs=+++
  Sum1 : Sum  Inputs=++|
  Supervisor : MATLAB Function  TreatAsAtomicUnit=on
      settings: PermitHierarchicalResolution=ParametersOnly
  Trigonometric Function : Trigonometry  Operator=tanh
  Qc : Outport
  wires:
  "T_d "/1 -> MATLAB Function/1(Td)
  [Rho] -> MATLAB Function/4(rho)
  [D] -> MATLAB Function/5(D)
  [eps_c] -> MATLAB Function/6(eps_c)
  MATLAB Function/2(T_r) -> Core controller/2("Tr ")
  MATLAB Function/1(n_d) -> Discrete Transfer Fcn/1
  Qff_0(nr)/1 -> Trigonometric Function/1
  Trigonometric Function/1 -> Qf_0/1
  NaN/1 -> Controller chosen/6
  Supervisor/1(u) -> Memory/1
  Memory/1 -> Controller chosen/1, Supervisor/1(control)
  Qff_1(nr)/1 -> Sum1/2
  Qf_0/1 -> Sum1/1
  [controller] -> Supervisor/2(input)
  Controller chosen/1 -> Sum/3
  Sum/1 -> Qc/1
  Core controller/2(Qcq) -> Controller chosen/3
  Core controller/3(Qcp) -> Controller chosen/4
  Core controller/4(Qcc) -> Controller chosen/5
  Core controller/1(Q_cn) -> Controller chosen/2
  [n_c] -> MATLAB Function/7(n_c)
  Discrete Derivative/1 -> Acceleration Limit/1
  Sum1/1 -> Sum/2
  Constant1/1 -> Discrete Transfer Fcn/2
  Constant2/1 -> Discrete Transfer Fcn/3
  Inertia compensation/1 -> Sum/1
  n/1 -> Core controller/3("n "), Supervisor/3(n)
  Acceleration Limit/1 -> Inertia compensation/1
  Discrete Transfer Fcn/1 -> Core controller/1(n_r), Delay/1, Qff_0(nr)/1, Qff_1(nr)/1, Discrete Derivative/1
  Delay/1 -> MATLAB Function/8(n_r)
  [Kt1r] -> MATLAB Function/3(K_t0r)
  [Kt1f] -> MATLAB Function/2(K_t0)

== system ctrl_TAPM_2015/Thruster control /Thruster 2/Propeller Hydrodynamics ==
  env : Inport
  n : Inport  Port=2
  Actual Force and Torque : MATLAB Function  TreatAsAtomicUnit=on
      settings: PermitHierarchicalResolution=ParametersOnly
  Ta : Outport
  Qa : Outport  Port=2
  wires:
  n/1 -> Actual Force and Torque/1(n)
  [D] -> Actual Force and Torque/7(D)
  [Kq2f] -> Actual Force and Torque/2(Kq)
  Actual Force and Torque/2(Qa) -> Qa/1
  [Rho] -> Actual Force and Torque/6(Rho)
  env/1 -> Actual Force and Torque/9(env)
  [Kt2f] -> Actual Force and Torque/3(Kt)
  Actual Force and Torque/1(Ta) -> Ta/1
  [Kt2r] -> Actual Force and Torque/4(Ktr)
  [Kq2r] -> Actual Force and Torque/5(Kqr)
  [eps_c] -> Actual Force and Torque/8(eps_c)

== system ctrl_TAPM_2015/Thruster control /Thruster 2/Shaft dynamics ==
  Qm : Inport
  Qa : Inport  Port=2
  Finding rotation speed : Gain  Gain=1/(2*pi*I_s)
  Integrator : Integrator  ExternalReset=either
  K_omega : Gain  Gain=K_omega*2*pi
  Sum : Sum  Inputs=-+-
  reset : S-Function  Priority=1  FunctionName=NIVeriStandIO  Parameters=width dtype portnum stime stype btype  SFunctionDeploymentMode=off  EnableBusSupport=off  mask(NI VeriStand Inport){portnum=1, width=-1, stime=-1, dtype=auto, stype=auto, btype=1}
      mask prompts: portnum "Port number:"; width "Port dimensions (-1 for dynamically sized):"; stime "Sample time (-1 for inherited):"; dtype "Data type:"; stype "Signal type:"; btype "Block type:"
      mask help: Use this inport on any level of nested subsystems to allow NI VeriStand software to map signals to it.
      mask init:
      | NIVeriStandIO_init;
      settings: CopyFcn=NIVeriStand_MDL_functions('', 'IO_copy');  DeleteFcn=NIVeriStand_MDL_functions('', 'IO_delete');  MoveFcn=set_param(gcb, 'Mask', 'on');
      mask Callback portnum: NIVeriStand_MDL_functions('', 'IO_setportnum');
      mask TypeOptions dtype: auto | double | single | int8 | uint8 | int16 | uint16 | int32 | uint32 | boolean
      mask Callback dtype: NIVeriStand_MDL_functions('', 'IO_booleansignal');
      mask TypeOptions stype: auto | real | complex
      mask Display:
      | patch([-x x], [-y y], [.90980 .81960 .32156]);
      | plot([xrad -x x xrad], [yrad -y y yrad]);
      | fprintf('NI In%d', portnum);
  n : Outport
  wires:
  Qm/1 -> Sum/2
  Sum/1 -> Finding rotation speed/1
  Qa/1 -> Sum/1
  K_omega/1 -> Sum/3
  Finding rotation speed/1 -> Integrator/1
  Integrator/1 -> K_omega/1, n/1
  reset/1 -> Integrator/2

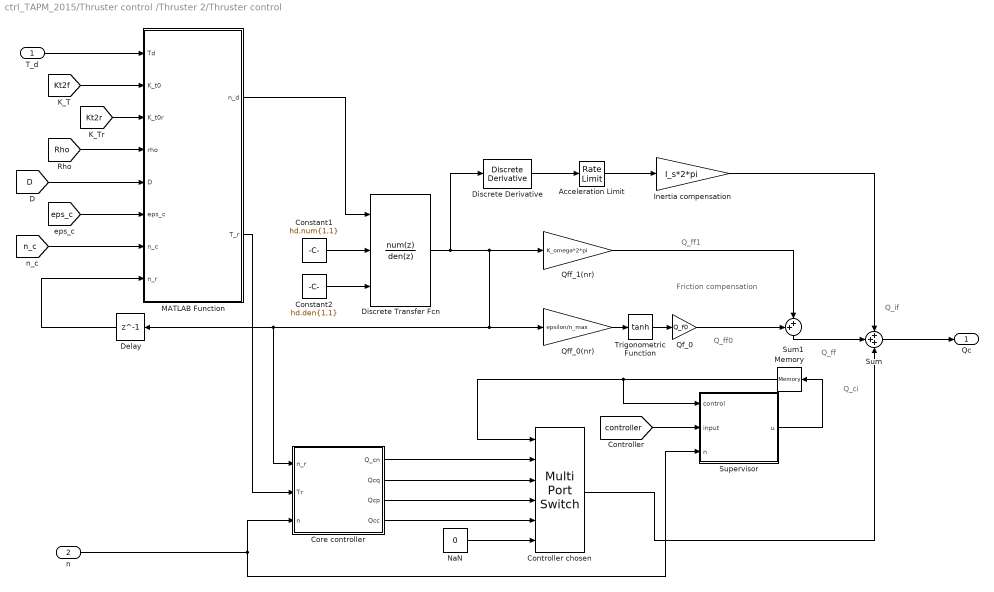
== system ctrl_TAPM_2015/Thruster control /Thruster 2/Thruster control ==
  note: Q_ci
  note: Q_if
  note: Q_ff
  note: Q_ff0
  note: Q_ff1
  note: Friction compensation
  "T_d " : Inport
  n : Inport  Port=2
  Acceleration Limit : RateLimiter  RisingSlewLimit=Max_Acceleration  FallingSlewLimit=-Max_Acceleration  SampleTimeMode=inherited
  Constant1 : Constant  Value=hd.num{1,1}  VectorParams1D=off
  Constant2 : Constant  Value=hd.den{1,1}  VectorParams1D=off
  Controller chosen : MultiPortSwitch  Inputs=5
  Core controller : Subsystem
  Delay : Delay  DelayLength=1  InitialCondition=0
  Discrete Transfer Fcn : DiscreteTransferFcn  NumeratorSource=Input port  Numerator=[8.76e-05 0.0003481 8.648e-05]  DenominatorSource=Input port  Denominator=[1 -1.974 0.9746]  SampleTime=0.01  a0EqualsOne=on
      settings: InputPortMap=u0,p1,p3
  Discrete Derivative : simulink/Discrete/Discrete Derivative  gainval=1.0  ICPrevScaledInput=0.0  InputProcessing=Inherited  OutMin=[]  OutMax=[]  OutDataType=fixdt(1, 16)  OutScaling=2^-10  DoSatur=off
  Inertia compensation : Gain  Gain=I_s*2*pi
  MATLAB Function : MATLAB Function  TreatAsAtomicUnit=on
      settings: PermitHierarchicalResolution=ParametersOnly
  Memory : Memory  X0=1
  NaN : Constant  Value=0
  Qf_0 : Gain  Gain=Q_f0
  Qff_0(nr) : Gain  Gain=epsilon/n_max
  Qff_1(nr) : Gain  Gain=K_omega*2*pi
  Sum : Sum  Inputs=+++
  Sum1 : Sum  Inputs=++|
  Supervisor : MATLAB Function  TreatAsAtomicUnit=on
      settings: PermitHierarchicalResolution=ParametersOnly
  Trigonometric Function : Trigonometry  Operator=tanh
  Qc : Outport
  wires:
  Sum/1 -> Qc/1
  MATLAB Function/2(T_r) -> Core controller/2("Tr ")
  Qff_0(nr)/1 -> Trigonometric Function/1
  Trigonometric Function/1 -> Qf_0/1
  Sum1/1 -> Sum/2
  Core controller/1(Q_cn) -> Controller chosen/2
  Core controller/4(Qcc) -> Controller chosen/5
  NaN/1 -> Controller chosen/6
  Memory/1 -> Supervisor/1(control), Controller chosen/1
  Qff_1(nr)/1 -> Sum1/2
  Qf_0/1 -> Sum1/1
  Controller chosen/1 -> Sum/3
  Inertia compensation/1 -> Sum/1
  Core controller/3(Qcp) -> Controller chosen/4
  Core controller/2(Qcq) -> Controller chosen/3
  [controller] -> Supervisor/2(input)
  "T_d "/1 -> MATLAB Function/1(Td)
  [Rho] -> MATLAB Function/4(rho)
  [D] -> MATLAB Function/5(D)
  [eps_c] -> MATLAB Function/6(eps_c)
  [n_c] -> MATLAB Function/7(n_c)
  Constant1/1 -> Discrete Transfer Fcn/2
  Constant2/1 -> Discrete Transfer Fcn/3
  MATLAB Function/1(n_d) -> Discrete Transfer Fcn/1
  Discrete Derivative/1 -> Acceleration Limit/1
  n/1 -> Supervisor/3(n), Core controller/3("n ")
  Discrete Transfer Fcn/1 -> Discrete Derivative/1, Qff_0(nr)/1, Core controller/1(n_r), Delay/1, Qff_1(nr)/1
  Acceleration Limit/1 -> Inertia compensation/1
  Supervisor/1(u) -> Memory/1
  Delay/1 -> MATLAB Function/8(n_r)
  [Kt2r] -> MATLAB Function/3(K_t0r)
  [Kt2f] -> MATLAB Function/2(K_t0)

== system ctrl_TAPM_2015/Thruster control /Thruster 3/Propeller Hydrodynamics ==
  env : Inport
  n : Inport  Port=2
  Actual Force and Torque : MATLAB Function  TreatAsAtomicUnit=on
      settings: PermitHierarchicalResolution=ParametersOnly
  Ta : Outport
  Qa : Outport  Port=2
  wires:
  n/1 -> Actual Force and Torque/1(n)
  [D] -> Actual Force and Torque/7(D)
  [Kq3f] -> Actual Force and Torque/2(Kq)
  Actual Force and Torque/2(Qa) -> Qa/1
  [Rho] -> Actual Force and Torque/6(Rho)
  env/1 -> Actual Force and Torque/9(env)
  [Kt3f] -> Actual Force and Torque/3(Kt)
  Actual Force and Torque/1(Ta) -> Ta/1
  [Kt3r] -> Actual Force and Torque/4(Ktr)
  [Kq3r] -> Actual Force and Torque/5(Kqr)
  [eps_c] -> Actual Force and Torque/8(eps_c)

== system ctrl_TAPM_2015/Thruster control /Thruster 3/Shaft dynamics ==
  Qm : Inport
  Qa : Inport  Port=2
  Finding rotation speed : Gain  Gain=1/(2*pi*I_s)
  Integrator : Integrator  ExternalReset=either
  K_omega : Gain  Gain=K_omega*2*pi
  Sum : Sum  Inputs=-+-
  reset : S-Function  Priority=1  FunctionName=NIVeriStandIO  Parameters=width dtype portnum stime stype btype  SFunctionDeploymentMode=off  EnableBusSupport=off  mask(NI VeriStand Inport){portnum=1, width=-1, stime=-1, dtype=auto, stype=auto, btype=1}
      mask prompts: portnum "Port number:"; width "Port dimensions (-1 for dynamically sized):"; stime "Sample time (-1 for inherited):"; dtype "Data type:"; stype "Signal type:"; btype "Block type:"
      mask help: Use this inport on any level of nested subsystems to allow NI VeriStand software to map signals to it.
      mask init:
      | NIVeriStandIO_init;
      settings: CopyFcn=NIVeriStand_MDL_functions('', 'IO_copy');  DeleteFcn=NIVeriStand_MDL_functions('', 'IO_delete');  MoveFcn=set_param(gcb, 'Mask', 'on');
      mask Callback portnum: NIVeriStand_MDL_functions('', 'IO_setportnum');
      mask TypeOptions dtype: auto | double | single | int8 | uint8 | int16 | uint16 | int32 | uint32 | boolean
      mask Callback dtype: NIVeriStand_MDL_functions('', 'IO_booleansignal');
      mask TypeOptions stype: auto | real | complex
      mask Display:
      | patch([-x x], [-y y], [.90980 .81960 .32156]);
      | plot([xrad -x x xrad], [yrad -y y yrad]);
      | fprintf('NI In%d', portnum);
  n : Outport
  wires:
  Qm/1 -> Sum/2
  Sum/1 -> Finding rotation speed/1
  Qa/1 -> Sum/1
  K_omega/1 -> Sum/3
  Finding rotation speed/1 -> Integrator/1
  Integrator/1 -> n/1, K_omega/1
  reset/1 -> Integrator/2

== system ctrl_TAPM_2015/Thruster control /Thruster 3/Thruster control ==
  note: Q_ci
  note: Q_if
  note: Q_ff
  note: Q_ff0
  note: Q_ff1
  note: Friction compensation
  "T_d " : Inport
  n : Inport  Port=2
  Acceleration limiter : RateLimiter  RisingSlewLimit=Max_Acceleration  FallingSlewLimit=-Max_Acceleration  SampleTimeMode=inherited
  Constant1 : Constant  Value=hd.num{1,1}  VectorParams1D=off
  Constant2 : Constant  Value=hd.den{1,1}  VectorParams1D=off
  Controller chosen : MultiPortSwitch  Inputs=5
  Core controller : Subsystem
  Delay : Delay  DelayLength=1  InitialCondition=0
  Discrete Transfer Fcn : DiscreteTransferFcn  NumeratorSource=Input port  Numerator=[8.76e-05 0.0003481 8.648e-05]  DenominatorSource=Input port  Denominator=[1 -1.974 0.9746]  SampleTime=0.01  a0EqualsOne=on
      settings: InputPortMap=u0,p1,p3
  Discrete Derivative : simulink/Discrete/Discrete Derivative  gainval=1.0  ICPrevScaledInput=0.0  InputProcessing=Inherited  OutMin=[]  OutMax=[]  OutDataType=fixdt(1, 16)  OutScaling=2^-10  DoSatur=off
  Inertia compensation : Gain  Gain=I_s*2*pi
  MATLAB Function : MATLAB Function  TreatAsAtomicUnit=on
      settings: PermitHierarchicalResolution=ParametersOnly
  Memory : Memory  X0=1
  NaN : Constant  Value=0
  Qf_0 : Gain  Gain=Q_f0
  Qff_0(nr) : Gain  Gain=epsilon/n_max
  Qff_1(nr) : Gain  Gain=K_omega*2*pi
  Sum : Sum  Inputs=+++
  Sum1 : Sum  Inputs=++|
  Supervisor : MATLAB Function  TreatAsAtomicUnit=on
      settings: PermitHierarchicalResolution=ParametersOnly
  Trigonometric Function : Trigonometry  Operator=tanh
  Qc : Outport
  wires:
  Sum/1 -> Qc/1
  MATLAB Function/2(T_r) -> Core controller/2("Tr ")
  Discrete Derivative/1 -> Acceleration limiter/1
  Qff_0(nr)/1 -> Trigonometric Function/1
  Trigonometric Function/1 -> Qf_0/1
  Sum1/1 -> Sum/2
  Core controller/1(Q_cn) -> Controller chosen/2
  Core controller/4(Qcc) -> Controller chosen/5
  NaN/1 -> Controller chosen/6
  Memory/1 -> Controller chosen/1, Supervisor/1(control)
  Qff_1(nr)/1 -> Sum1/2
  Qf_0/1 -> Sum1/1
  Controller chosen/1 -> Sum/3
  Inertia compensation/1 -> Sum/1
  Core controller/3(Qcp) -> Controller chosen/4
  Core controller/2(Qcq) -> Controller chosen/3
  [controller] -> Supervisor/2(input)
  "T_d "/1 -> MATLAB Function/1(Td)
  [Rho] -> MATLAB Function/4(rho)
  [D] -> MATLAB Function/5(D)
  [eps_c] -> MATLAB Function/6(eps_c)
  [n_c] -> MATLAB Function/7(n_c)
  Constant1/1 -> Discrete Transfer Fcn/2
  Constant2/1 -> Discrete Transfer Fcn/3
  MATLAB Function/1(n_d) -> Discrete Transfer Fcn/1
  n/1 -> Supervisor/3(n), Core controller/3("n ")
  Discrete Transfer Fcn/1 -> Discrete Derivative/1, Core controller/1(n_r), Delay/1, Qff_0(nr)/1, Qff_1(nr)/1
  Acceleration limiter/1 -> Inertia compensation/1
  Supervisor/1(u) -> Memory/1
  Delay/1 -> MATLAB Function/8(n_r)
  [Kt3f] -> MATLAB Function/3(K_t0r)
  [Kt3f] -> MATLAB Function/2(K_t0)

== system ctrl_TAPM_2015/Thruster control /Thruster 4/Propeller Hydrodynamics ==
  env : Inport
  n : Inport  Port=2
  Actual Force and Torque : MATLAB Function  TreatAsAtomicUnit=on
      settings: PermitHierarchicalResolution=ParametersOnly
  Ta : Outport
  Qa : Outport  Port=2
  wires:
  n/1 -> Actual Force and Torque/1(n)
  [D] -> Actual Force and Torque/7(D)
  [Kq4f] -> Actual Force and Torque/2(Kq)
  Actual Force and Torque/2(Qa) -> Qa/1
  [Rho] -> Actual Force and Torque/6(Rho)
  env/1 -> Actual Force and Torque/9(env)
  [Kt4f] -> Actual Force and Torque/3(Kt)
  Actual Force and Torque/1(Ta) -> Ta/1
  [Kt4r] -> Actual Force and Torque/4(Ktr)
  [Kq4r] -> Actual Force and Torque/5(Kqr)
  [eps_c] -> Actual Force and Torque/8(eps_c)

== system ctrl_TAPM_2015/Thruster control /Thruster 4/Shaft dynamics ==
  Qm : Inport
  Qa : Inport  Port=2
  Finding rotation speed : Gain  Gain=1/(2*pi*I_s)
  Integrator : Integrator  ExternalReset=either
  K_omega : Gain  Gain=K_omega*2*pi
  Sum : Sum  Inputs=-+-
  reset : S-Function  Priority=1  FunctionName=NIVeriStandIO  Parameters=width dtype portnum stime stype btype  SFunctionDeploymentMode=off  EnableBusSupport=off  mask(NI VeriStand Inport){portnum=1, width=-1, stime=-1, dtype=auto, stype=auto, btype=1}
      mask prompts: portnum "Port number:"; width "Port dimensions (-1 for dynamically sized):"; stime "Sample time (-1 for inherited):"; dtype "Data type:"; stype "Signal type:"; btype "Block type:"
      mask help: Use this inport on any level of nested subsystems to allow NI VeriStand software to map signals to it.
      mask init:
      | NIVeriStandIO_init;
      settings: CopyFcn=NIVeriStand_MDL_functions('', 'IO_copy');  DeleteFcn=NIVeriStand_MDL_functions('', 'IO_delete');  MoveFcn=set_param(gcb, 'Mask', 'on');
      mask Callback portnum: NIVeriStand_MDL_functions('', 'IO_setportnum');
      mask TypeOptions dtype: auto | double | single | int8 | uint8 | int16 | uint16 | int32 | uint32 | boolean
      mask Callback dtype: NIVeriStand_MDL_functions('', 'IO_booleansignal');
      mask TypeOptions stype: auto | real | complex
      mask Display:
      | patch([-x x], [-y y], [.90980 .81960 .32156]);
      | plot([xrad -x x xrad], [yrad -y y yrad]);
      | fprintf('NI In%d', portnum);
  n : Outport
  wires:
  Qm/1 -> Sum/2
  Sum/1 -> Finding rotation speed/1
  Qa/1 -> Sum/1
  K_omega/1 -> Sum/3
  Finding rotation speed/1 -> Integrator/1
  Integrator/1 -> K_omega/1, n/1
  reset/1 -> Integrator/2

== system ctrl_TAPM_2015/Thruster control /Thruster 4/Thruster control ==
  note: Q_ci
  note: Q_if
  note: Q_ff
  note: Q_ff0
  note: Q_ff1
  note: Friction compensation
  "T_d " : Inport
  n : Inport  Port=2
  Acceleration limiter : RateLimiter  RisingSlewLimit=Max_Acceleration  FallingSlewLimit=-Max_Acceleration  SampleTimeMode=inherited
  Constant1 : Constant  Value=hd.num{1,1}  VectorParams1D=off
  Constant2 : Constant  Value=hd.den{1,1}  VectorParams1D=off
  Controller chosen : MultiPortSwitch  Inputs=5
  Core controller : Subsystem
  Delay : Delay  DelayLength=1  InitialCondition=0
  Discrete Transfer Fcn : DiscreteTransferFcn  NumeratorSource=Input port  Numerator=[8.76e-05 0.0003481 8.648e-05]  DenominatorSource=Input port  Denominator=[1 -1.974 0.9746]  SampleTime=0.01  a0EqualsOne=on
      settings: InputPortMap=u0,p1,p3
  Discrete Derivative : simulink/Discrete/Discrete Derivative  gainval=1.0  ICPrevScaledInput=0.0  InputProcessing=Inherited  OutMin=[]  OutMax=[]  OutDataType=fixdt(1, 16)  OutScaling=2^-10  DoSatur=off
  Inertia compensation : Gain  Gain=I_s*2*pi
  MATLAB Function : MATLAB Function  TreatAsAtomicUnit=on
      settings: PermitHierarchicalResolution=ParametersOnly
  Memory : Memory  X0=1
  NaN : Constant  Value=0
  Qf_0 : Gain  Gain=Q_f0
  Qff_0(nr) : Gain  Gain=epsilon/n_max
  Qff_1(nr) : Gain  Gain=K_omega*2*pi
  Sum : Sum  Inputs=+++
  Sum1 : Sum  Inputs=++|
  Supervisor : MATLAB Function  TreatAsAtomicUnit=on
      settings: PermitHierarchicalResolution=ParametersOnly
  Trigonometric Function : Trigonometry  Operator=tanh
  Qc : Outport
  wires:
  Sum/1 -> Qc/1
  MATLAB Function/2(T_r) -> Core controller/2("Tr ")
  Discrete Derivative/1 -> Acceleration limiter/1
  Qff_0(nr)/1 -> Trigonometric Function/1
  Trigonometric Function/1 -> Qf_0/1
  Sum1/1 -> Sum/2
  Core controller/1(Q_cn) -> Controller chosen/2
  Core controller/4(Qcc) -> Controller chosen/5
  NaN/1 -> Controller chosen/6
  Memory/1 -> Controller chosen/1, Supervisor/1(control)
  Qff_1(nr)/1 -> Sum1/2
  Qf_0/1 -> Sum1/1
  Controller chosen/1 -> Sum/3
  Inertia compensation/1 -> Sum/1
  Core controller/3(Qcp) -> Controller chosen/4
  Core controller/2(Qcq) -> Controller chosen/3
  [controller] -> Supervisor/2(input)
  "T_d "/1 -> MATLAB Function/1(Td)
  [Rho] -> MATLAB Function/4(rho)
  [D] -> MATLAB Function/5(D)
  [eps_c] -> MATLAB Function/6(eps_c)
  [n_c] -> MATLAB Function/7(n_c)
  Constant1/1 -> Discrete Transfer Fcn/2
  Constant2/1 -> Discrete Transfer Fcn/3
  MATLAB Function/1(n_d) -> Discrete Transfer Fcn/1
  n/1 -> Supervisor/3(n), Core controller/3("n ")
  Discrete Transfer Fcn/1 -> Discrete Derivative/1, Core controller/1(n_r), Delay/1, Qff_0(nr)/1, Qff_1(nr)/1
  Acceleration limiter/1 -> Inertia compensation/1
  Supervisor/1(u) -> Memory/1
  Delay/1 -> MATLAB Function/8(n_r)
  [Kt4r] -> MATLAB Function/3(K_t0r)
  [Kt4f] -> MATLAB Function/2(K_t0)
